simulink model "ImpedanceControl"  (R2023b)
settings: Solver=VariableStepAuto  StartTime=0.0  StopTime=10.0  RelTol=1e-3
settings Model: Creator=91996  LastModifiedBy=91996

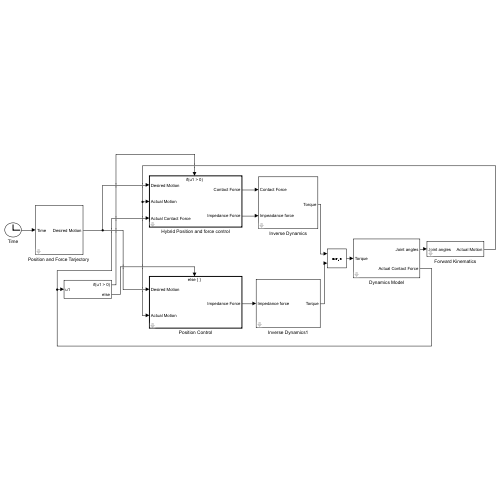
[thumbnail: Simulink's stored preview of the top-level diagram]
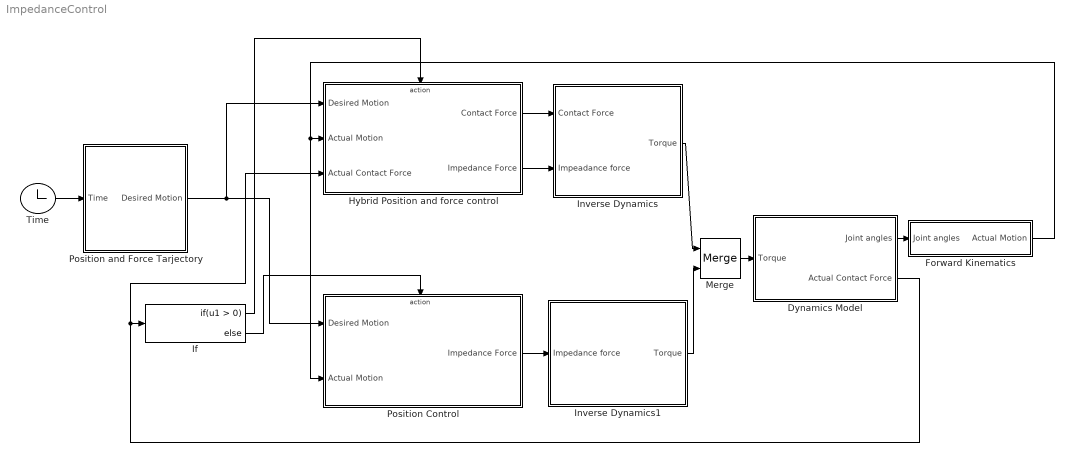
== system ImpedanceControl ==
  Dynamics Model : Subsystem
      mask DialogControl C Prompt: Parameters
  Forward Kinematics : Subsystem
      mask DialogControl Kinematics Prompt: Parameters
  Hybrid Position and force control : Subsystem
      mask DialogControl A Prompt: Parameters
  If : If
  Inverse Dynamics : Subsystem
      mask DialogControl B Prompt: Parameters
  Inverse Dynamics1 : Subsystem
      mask DialogControl B Prompt: Parameters
  Merge : Merge
  Position Control : Subsystem
      mask DialogControl A Prompt: Parameters
  "Position and Force Tarjectory " : Subsystem
      mask DialogControl E Prompt: Parameters
  Time : Clock
  wires:
  "Position and Force Tarjectory "/1(Desired Motion) -> Hybrid Position and force control/1(Desired Motion), Position Control/1(Desired Motion)
  Time/1 -> "Position and Force Tarjectory "/1(Time)
  Forward Kinematics/1(Actual Motion) -> Position Control/2(Actual Motion), Hybrid Position and force control/2(Actual Motion)
  Dynamics Model/1(Joint angles) -> Forward Kinematics/1(Joint angles)
  Hybrid Position and force control/1(Contact Force) -> Inverse Dynamics/1(Contact Force)
  Hybrid Position and force control/2(Impedance Force) -> Inverse Dynamics/2(Impeadance force)
  Dynamics Model/2(Actual Contact Force) -> Hybrid Position and force control/3(Actual Contact Force), If/1
  If/1 -> Hybrid Position and force control/Action
  If/2 -> Position Control/Action
  Position Control/1(Impedance Force) -> Inverse Dynamics1/1(Impedance force)
  Merge/1 -> Dynamics Model/1(Torque)
  Inverse Dynamics1/1(Torque) -> Merge/2
  Inverse Dynamics/1(Torque) -> Merge/1

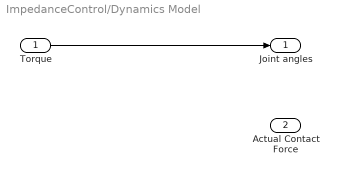
== system ImpedanceControl/Dynamics Model ==
  Torque : Inport
  Joint angles : Outport
  Actual Contact Force : Outport  Port=2
  wires:
  Torque/1 -> Joint angles/1

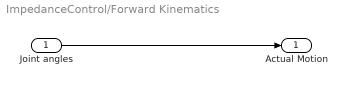
== system ImpedanceControl/Forward Kinematics ==
  Joint angles : Inport
  Actual Motion : Outport
  wires:
  Joint angles/1 -> Actual Motion/1

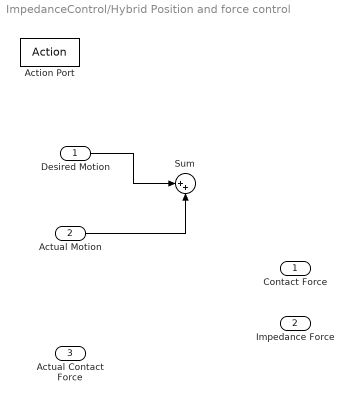
== system ImpedanceControl/Hybrid Position and force control ==
  Desired Motion : Inport
  Actual Motion : Inport  Port=2
  Actual Contact Force : Inport  Port=3
  Action Port : ActionPort  ActionPortLabel=if(u1 > 0)
  Sum : Sum  Inputs=|++
  Contact Force : Outport
  Impedance Force : Outport  Port=2
  wires:
  Desired Motion/1 -> Sum/1
  Actual Motion/1 -> Sum/2

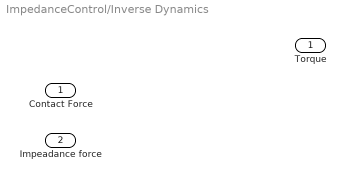
== system ImpedanceControl/Inverse Dynamics ==
  Contact Force : Inport
  Impeadance force : Inport  Port=2
  Torque : Outport
  wires:
  ? -> Torque/1

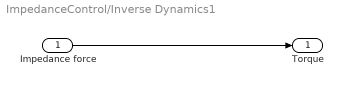
== system ImpedanceControl/Inverse Dynamics1 ==
  Impedance force : Inport
  Torque : Outport
  wires:
  Impedance force/1 -> Torque/1

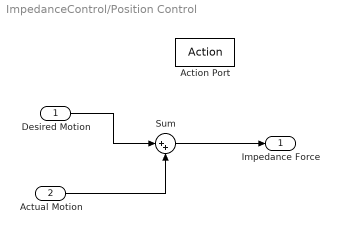
== system ImpedanceControl/Position Control ==
  Desired Motion : Inport
  Actual Motion : Inport  Port=2
  Action Port : ActionPort  ActionPortLabel=else
  Sum : Sum  Inputs=|++
  Impedance Force : Outport
  wires:
  Desired Motion/1 -> Sum/1
  Actual Motion/1 -> Sum/2
  Sum/1 -> Impedance Force/1

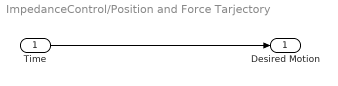
== system ImpedanceControl/Position and Force Tarjectory  ==
  Time : Inport
  Desired Motion : Outport
  wires:
  Time/1 -> Desired Motion/1
